simulink model "malith10"  (R2016a)
settings: Solver=VariableStepAuto  StartTime=0.0  StopTime=20  RelTol=1e-3
libraries: powerlib_meascontrol x7, powerlib x5, simulink x1
settings Model: Creator=malit  LastModifiedBy=malit
settings SolverCC: ZeroCrossAlgorithm=Adaptive

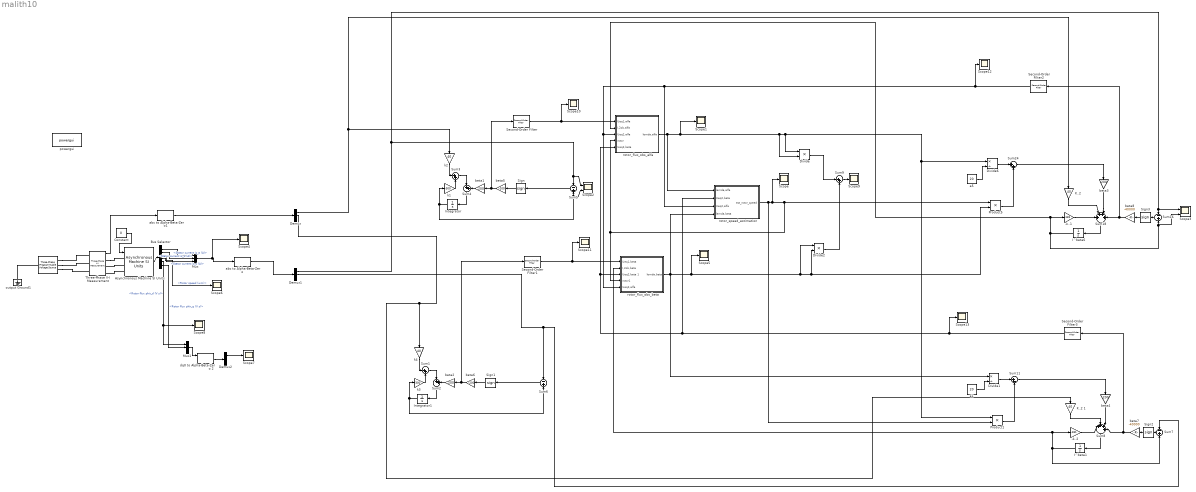
== system malith10 ==
  " " : powerlib/Electrical Sources/Three-Phase Programmable Voltage Source  PositiveSequence="[460 0  60]"  VariationEntity=Frequency  VariationType=Step  VariationTypeAlt=Step  VariationStep=100  VariationRate=10  VariationMagnitude=0.3  VariationFrequency=2  VariationTiming=[3 8]  VariationPhaseA=off  Amplitudes=[1 0.8 1.2 1.0]  TimeValues=[0 0.1 0.15 0.2]  HarmonicGeneration=off  HarmonicA=[5 0.08 -45 2]  HarmonicB=[2 0 0 2]  Timing="[0.1  1]"  BusType=swing  Pref=0  Qref=0  Qmin=-inf  Qmax=inf
  -k..1 : Gain  Gain=-181
  -k..2 : Gain  Gain=-181
  Asynchronous Machine SI Units : powerlib/Machines/Asynchronous Machine SI Units  RotorType=Squirrel-cage  PresetModel=No  MechanicalLoad=Torque Tm  ShowDetailedParameters=on  ReferenceFrame=Stationary  Units=SI  MeasurementBus=off  NominalParameters=[3730 460 60]  Stator=[1.115 0.005974]  Rotor=[1.083 0.005974]  Cage1=[0.4155 0.002066]  Cage2=[0.4168 0.0003495]  Lm=0.2037  Mechanical=[0.02 0.005752 2]  PolePairs=2  InitialConditions=[0 0 0 0 0 0 0 0]  SimulateSaturation=off  Saturation=[14.03593122, 27.81365428, 53.79336849, 72.68890987, 97.98006896, 148.6815601, 215.7428561, 302.9841135, 428.7778367 ; 230, 322, 414, 460, 506, 552, 598, 644, 690]  LoadFlowParameters=1492000  TsPowergui=0  TsBlock=-1  IterativeModel=Trapezoidal non iterative  IterativeDiscreteModel=Trapezoidal non iterative  Pmec=1.492e+006
  Bus Selector : BusSelector  OutputSignals=Stator measurements.Stator current is_a (A),Stator measurements.Stator current is_b (A),Stator measurements.Stator current is_c (A),Mechanical.Rotor speed (wm),Rotor measurements.Rotor flux phir_d (V s),Rotor measurements.Rotor flux phir_q (V s)
  Constant : Constant  Value=0
  Demux : Demux  Outputs=3
  Demux1 : Demux  Outputs=3
  Demux2 : Demux  Outputs=3
  Divide : Product  Inputs=**
  Divide1 : Product  Inputs=*/
  Divide2 : Product  Inputs=**
  Divide6 : Product  Inputs=*/
  I^beta1 : Integrator
  I^beta6 : Integrator
  Integrator : Integrator
  Integrator1 : Integrator
  "K..2 " : Gain  Gain=40
  K..2 1 : Gain  Gain=40
  Mux : Mux  Inputs=3
  Mux1 : Mux  Inputs=3
  Product1 : Product
  Product5 : Product
  Scope{,1,4..13} (12 alike) : Scope
  Scope2 : Scope  NumInputPorts=2
  Scope3 : Scope  NumInputPorts=2
  Second-Order Filter{,1..3} (4 alike) : powerlib_meascontrol/Filters/Second-Order Filter  FilterType=Bandpass  Fo=120  Zeta=0.707  Ts=0  Initialize=on  Vac_Init="[0,  0,  60]"  Vdc_Init=0  PlotResponse=off  FreqRange=[0, 500, 1]
  Sign{,1..3} (4 alike) : Signum
  Sum{1..4,9,24} (6 alike) : Sum  Inputs=|++
  Sum11 : Sum  Inputs=|+-
  Sum{5..7,16} (4 alike) : Sum  Inputs=-+
  Sum18 : Sum  Inputs=++++
  Sum8 : Sum  Inputs=|++++
  Three-Phase V-I Measurement : powerlib/Measurements/Three-Phase V-I Measurement  VoltageMeasurement=phase-to-ground  SetLabelV=off  LabelV=Vabc  Vpu=off  VpuLL=off  CurrentMeasurement=no  SetLabelI=off  LabelI=Iabc  Ipu=off  Pbase=100e6  Vbase=500e3  OutputType=Complex  PhasorSimulation=off  PSBequivalent=0
  a1 : Constant  Value=20
  a5 : Constant  Value=20
  abc to Alpha-Beta-Zero : powerlib_meascontrol/Transformations/abc to Alpha-Beta-Zero
  abc to Alpha-Beta-Zero1 : powerlib_meascontrol/Transformations/abc to Alpha-Beta-Zero
  beta{1..4} (4 alike) : Gain  Gain=200
  beta5 : Gain  Gain=-200
  beta6 : Gain  Gain=-200
  beta7 : Gain  Gain=-40000
  beta8 : Gain  Gain=-40000
  dq0 to Alpha-Beta-Zero 2 : powerlib_meascontrol/Transformations/dq0 to Alpha-Beta-Zero  Alignment=Aligned with phase A axis
  k1 : Gain  Gain=-300
  k2 : Gain  Gain=40
  k3 : Gain  Gain=-300
  k4 : Gain  Gain=40
  output Ground1 : powerlib/Elements/Ground  LConnTagsString=a
  powergui : powerlib/powergui  Priority=2  SimulationMode=Discrete  SolverType=Tustin/Backward Euler (TBE)  SampleTime=50e-7  frequency=60  SPID=off  DisableSnubberDevices=off  DisableRonSwitches=off  DisableVfSwitches=off  SwTol=0  DisplayEquations=off  Interpol=off  ExternalGateDelay=off  methode=off  Ts=0  FunctionMessages=off  echomessages=off  HookPort=off  EnableUseOfTLC=off  x0status=blocks  frequencyindice=60  Pbase=100e6  ErrMax=0.0001  Iterations=50  UnitsV=kV  UnitsW=MW  buscounter=0  RestoreLinks=warning  ResistiveCurrentMeasurement=off  Frange=0:0.5:500  Ylog=off  Xlog=off  ShowGrid=off  save=on  variable=Zmes  structure=0  ZoomFFT=on  StartTime=0.0  cycles=1  DisplayStyle=off  fundamental=60  FreqAxis=off  MaxFrequency=1000  frequencyindicesteady=1  RmsSteady=1  display=off
  rotor_flux_obs_alfa : Subsystem
  rotor_flux_obs_beta : Subsystem
  rotor_speed_estimation : Subsystem
  wires:
  I^beta6/1 -> rotor_flux_obs_alfa/2(I,2ob,alfa), -k..1/1, Scope3/2, Sum16/2
  Sum16/1 -> Sign3/1
  Sum24/1 -> beta3/1
  rotor_flux_obs_alfa/1(lemda,alfa) -> Scope1/1, Divide/2, Divide/1, Product1/1, Divide6/1, rotor_speed_estimation/1(lemda,alfa)
  a5/1 -> Divide6/2
  Divide6/1 -> Sum24/1
  Product5/1 -> Sum24/2
  rotor_flux_obs_beta/1(lemda,beta) -> rotor_speed_estimation/4(lemda,beta), Divide1/1, Scope5/1, Divide2/1, Divide2/2, Product5/2
  -k..2/1 -> Sum8/1
  Sum7/1 -> Sign2/1
  Sum11/1 -> beta4/1
  a1/1 -> Divide1/2
  Divide1/1 -> Sum11/1
  Product1/1 -> Sum11/2
  I^beta1/1 -> rotor_flux_obs_beta/2(I,2ob,beta), -k..2/1, Sum7/2
  Demux/1 -> k2/1, "K..2 "/1
  Demux/2 -> k4/1, K..2 1/1
  Demux1/2 -> Sum6/1, Sum7/1
  Asynchronous Machine SI Units/1 -> Bus Selector/1
  Bus Selector/1 -> Mux/1  "<Stator current is_a (A)>"
  Bus Selector/3 -> Mux/3  "<Stator current is_c (A)>"
  Bus Selector/2 -> Mux/2  "<Stator current is_b (A)>"
  Mux/1 -> Scope4/1, abc to Alpha-Beta-Zero/1
  abc to Alpha-Beta-Zero1/1 -> Demux/1
  abc to Alpha-Beta-Zero/1 -> Demux1/1
  Constant/1 -> Asynchronous Machine SI Units/1
  k1/1 -> Sum3/2
  Sum3/1 -> Sum4/1
  k2/1 -> Sum3/1
  Sum4/1 -> Integrator/1
  beta1/1 -> Sum4/2
  Integrator/1 -> Scope2/2, Sum5/2, k1/1
  Sum5/1 -> Sign/1
  Sign/1 -> beta5/1
  k3/1 -> Sum1/2
  Sum1/1 -> Sum2/1
  k4/1 -> Sum1/1
  Sum2/1 -> Integrator1/1
  beta2/1 -> Sum2/2
  Integrator1/1 -> Sum6/2, k3/1
  Sum6/1 -> Sign1/1
  Sign1/1 -> beta6/1
  Sign2/1 -> beta7/1
  Sign3/1 -> beta8/1
  Sum8/1 -> I^beta1/1
  K..2 1/1 -> Sum8/2
  beta4/1 -> Sum8/3
  beta3/1 -> Sum18/3
  "K..2 "/1 -> Sum18/2
  -k..1/1 -> Sum18/1
  Sum18/1 -> I^beta6/1
  Demux1/1 -> Scope2/1, Sum5/1, Scope3/1, Sum16/1
  Bus Selector/4 -> Scope6/1  "<Rotor speed (wm)>"
  beta5/1 -> Second-Order Filter/1, beta1/1
  beta6/1 -> Second-Order Filter1/1, beta2/1
  beta8/1 -> Second-Order Filter2/1, Sum18/4
  beta7/1 -> Second-Order Filter3/1, Sum8/4
  Three-Phase V-I Measurement/1 -> abc to Alpha-Beta-Zero1/1
  Mux1/1 -> dq0 to Alpha-Beta-Zero 2/1
  dq0 to Alpha-Beta-Zero 2/1 -> Demux2/1
  Demux2/1 -> Scope7/1
  Bus Selector/5 -> Scope8/1, Mux1/1  "<Rotor flux phir_d (V s)>"
  Bus Selector/6 -> Mux1/2  "<Rotor flux phir_q (V s)>"
  rotor_speed_estimation/1(est_rotor_speed) -> Product5/1, rotor_flux_obs_beta/4(rotor1), rotor_flux_obs_alfa/4(rotor), Scope/1, Product1/2
  Divide2/1 -> Sum9/2
  Divide/1 -> Sum9/1
  Sum9/1 -> Scope9/1
  Second-Order Filter/1 -> Scope10/1, rotor_flux_obs_alfa/1("Ueq1,alfa ")
  Second-Order Filter1/1 -> Scope11/1, rotor_flux_obs_beta/1("Ueq1,beta ")
  Second-Order Filter2/1 -> Scope12/1, rotor_speed_estimation/3(Ueq2,alfa), rotor_flux_obs_beta/5("Ueq2,alfa "), rotor_flux_obs_alfa/3("Ueq2,alfa ")
  Second-Order Filter3/1 -> Scope13/1, rotor_flux_obs_beta/3(Ueq2,beta 1), rotor_flux_obs_alfa/5("Ueq2,beta "), rotor_speed_estimation/2(Ueq2,beta)
  connections:
  " "/RConn1 -- Three-Phase V-I Measurement/LConn1
  " "/RConn2 -- Three-Phase V-I Measurement/LConn2
  " "/RConn3 -- Three-Phase V-I Measurement/LConn3
  Three-Phase V-I Measurement/RConn1 -- Asynchronous Machine SI Units/LConn1
  Asynchronous Machine SI Units/LConn2 -- Three-Phase V-I Measurement/RConn2
  Asynchronous Machine SI Units/LConn3 -- Three-Phase V-I Measurement/RConn3
  " "/LConn1 -- output Ground1/LConn1

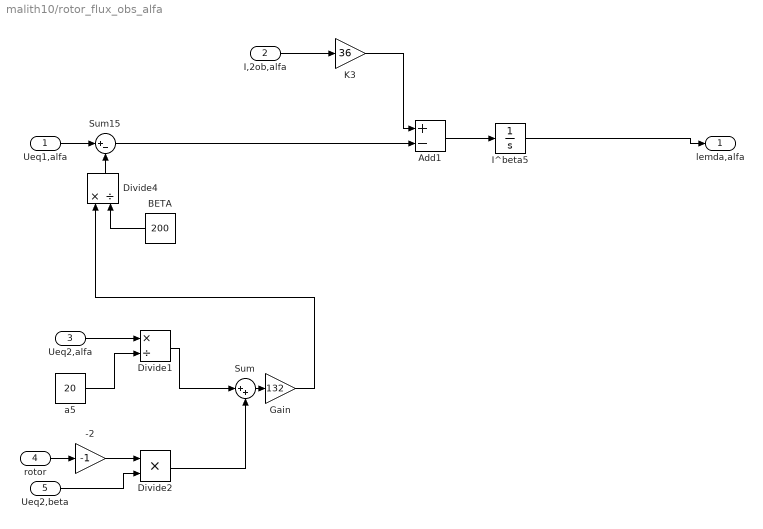
== system malith10/rotor_flux_obs_alfa ==
  "Ueq1,alfa " : Inport
  I,2ob,alfa : Inport  Port=2
  "Ueq2,alfa " : Inport  Port=3
  rotor : Inport  Port=4
  "Ueq2,beta " : Inport  Port=5
  -2 : Gain  Gain=-1
  Add1 : Sum  Inputs=+-
  BETA : Constant  Value=200
  Divide1 : Product  Inputs=*/
  Divide2 : Product  Inputs=**
  Divide4 : Product  Inputs=*/
  Gain : Gain  Gain=132
  I^beta5 : Integrator
  "K3 " : Gain  Gain=36
  Sum : Sum  Inputs=|++
  Sum15 : Sum  Inputs=|+-
  a5 : Constant  Value=20
  lemda,alfa : Outport
  wires:
  "K3 "/1 -> Add1/1
  Sum15/1 -> Add1/2
  Divide4/1 -> Sum15/2
  BETA/1 -> Divide4/2
  Add1/1 -> I^beta5/1
  "Ueq1,alfa "/1 -> Sum15/1
  "Ueq2,alfa "/1 -> Divide1/1
  I,2ob,alfa/1 -> "K3 "/1
  a5/1 -> Divide1/2
  rotor/1 -> -2/1
  -2/1 -> Divide2/1
  "Ueq2,beta "/1 -> Divide2/2
  Divide1/1 -> Sum/1
  Divide2/1 -> Sum/2
  Sum/1 -> Gain/1
  Gain/1 -> Divide4/1
  I^beta5/1 -> lemda,alfa/1

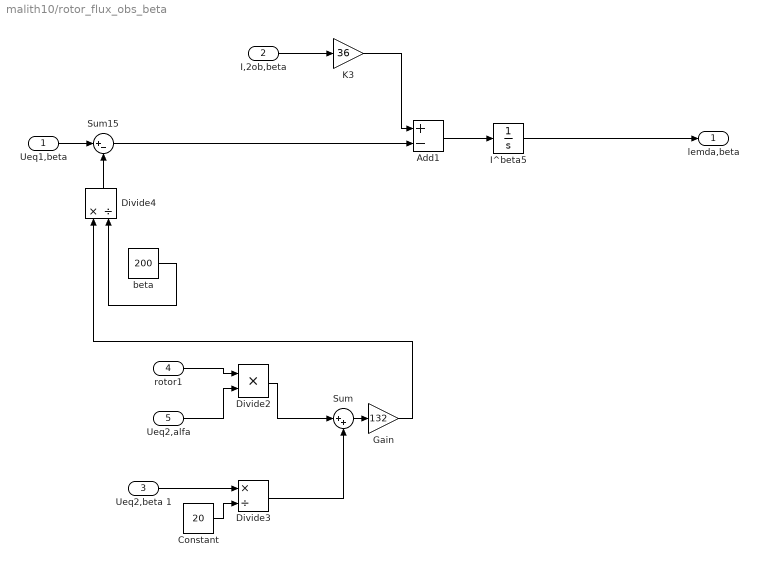
== system malith10/rotor_flux_obs_beta ==
  "Ueq1,beta " : Inport
  I,2ob,beta : Inport  Port=2
  Ueq2,beta 1 : Inport  Port=3
  rotor1 : Inport  Port=4
  "Ueq2,alfa " : Inport  Port=5
  Add1 : Sum  Inputs=+-
  Constant : Constant  Value=20
  Divide2 : Product  Inputs=**
  Divide3 : Product  Inputs=*/
  Divide4 : Product  Inputs=*/
  Gain : Gain  Gain=132
  I^beta5 : Integrator
  "K3 " : Gain  Gain=36
  Sum : Sum  Inputs=|++
  Sum15 : Sum  Inputs=|+-
  beta : Constant  Value=200
  lemda,beta : Outport
  wires:
  "K3 "/1 -> Add1/1
  Sum15/1 -> Add1/2
  Add1/1 -> I^beta5/1
  "Ueq1,beta "/1 -> Sum15/1
  I,2ob,beta/1 -> "K3 "/1
  rotor1/1 -> Divide2/1
  "Ueq2,alfa "/1 -> Divide2/2
  Divide2/1 -> Sum/1
  Divide3/1 -> Sum/2
  Sum/1 -> Gain/1
  Ueq2,beta 1/1 -> Divide3/1
  Constant/1 -> Divide3/2
  Gain/1 -> Divide4/1
  Divide4/1 -> Sum15/2
  beta/1 -> Divide4/2
  I^beta5/1 -> lemda,beta/1

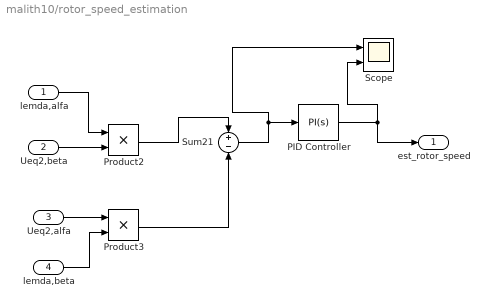
== system malith10/rotor_speed_estimation ==
  lemda,alfa : Inport
  Ueq2,beta : Inport  Port=2
  Ueq2,alfa : Inport  Port=3
  lemda,beta : Inport  Port=4
  PID Controller : simulink/Continuous/PID Controller  Controller=PI  TimeDomain=Continuous-time  SampleTime=-1  IntegratorMethod=Forward Euler  FilterMethod=Forward Euler  Form=Ideal  UseFilter=on  ControllerParametersSource=internal  P=0.001  I=20  D=0  N=100  InitialConditionSource=internal  InitialConditionForIntegrator=0  InitialConditionForFilter=0  ExternalReset=none  ZeroCross=off  LimitOutput=off  UpperSaturationLimit=inf  LowerSaturationLimit=-inf  LinearizeAsGain=on  AntiWindupMode=none  Kb=1  TrackingMode=off  Kt=1  PParamMin=[]  PParamMax=[]  IParamMin=[]  IParamMax=[]  DParamMin=[]  DParamMax=[]  NParamMin=[]  NParamMax=[]  KbParamMin=[]  KbParamMax=[]  KtParamMin=[]  KtParamMax=[]  POutMin=[]  POutMax=[]  IOutMin=[]  IOutMax=[]  DOutMin=[]  DOutMax=[]  NOutMin=[]  NOutMax=[]  KbOutMin=[]  KbOutMax=[]  KtOutMin=[]  KtOutMax=[]  IntegratorOutMin=[]  IntegratorOutMax=[]  FilterOutMin=[]  FilterOutMax=[]  SumOutMin=[]  SumOutMax=[]  SumI1OutMin=[]  SumI1OutMax=[]  SumI2OutMin=[]  SumI2OutMax=[]  SumI3OutMin=[]  SumI3OutMax=[]  SumDOutMin=[]  SumDOutMax=[]  SaturationOutMin=[]  SaturationOutMax=[]  IntegratorContinuousStateAttributes=''  IntegratorStateMustResolveToSignalObject=off  IntegratorRTWStateStorageClass=Auto  FilterContinuousStateAttributes=''  FilterStateMustResolveToSignalObject=off  FilterRTWStateStorageClass=Auto  DifferentiatorICPrevScaledInput=0  DifferentiatorOutMin=[]  DifferentiatorOutMax=[]
  Product2 : Product
  Product3 : Product
  Scope : Scope  NumInputPorts=2
  Sum21 : Sum  Inputs=+-
  est_rotor_speed : Outport
  wires:
  Ueq2,alfa/1 -> Product3/1
  lemda,alfa/1 -> Product2/1
  Product3/1 -> Sum21/2
  lemda,beta/1 -> Product3/2
  Ueq2,beta/1 -> Product2/2
  Sum21/1 -> PID Controller/1, Scope/1
  Product2/1 -> Sum21/1
  PID Controller/1 -> est_rotor_speed/1, Scope/2
